simulink model "System_discrete_RST"  (R2020a)
settings: Solver=FixedStepAuto  StartTime=0.0  StopTime=30  RelTol=1e-3
values from neighbouring files (symbols this model uses):
  Te = 1e-3    (= 0.001)    [CommandeMCC.m]
undefined symbols (not defined in the file or in its folder): Amat, Bmat, ConsPolDen, ConsPolNum, RetPolDen, RetPolNum, SatPolDen, SatPolNum
libraries: simulink x1
settings Model: Creator=antoi  LastModifiedBy=antoi
settings OptimizationCC: OptimizeBlockIOStorage=off  OptimizeDataStoreBuffers=off  BusAssignmentInplaceUpdate=off
settings DebuggingCC: SFUnexpectedBacktrackingDiag=warning  SFNoUnconditionalDefaultTransitionDiag=warning
settings RTWCC: GenerateReport=on  BuildConfiguration=Debug  LaunchReport=on
settings CodeAppCC: ForceParamTrailComments=on  MATLABSourceComments=on  EnableCustomComments=on
settings GRTTargetCC: CombineSignalStateStructs=on  SupportVariableSizeSignals=on  MultiInstanceErrorCode=Warning

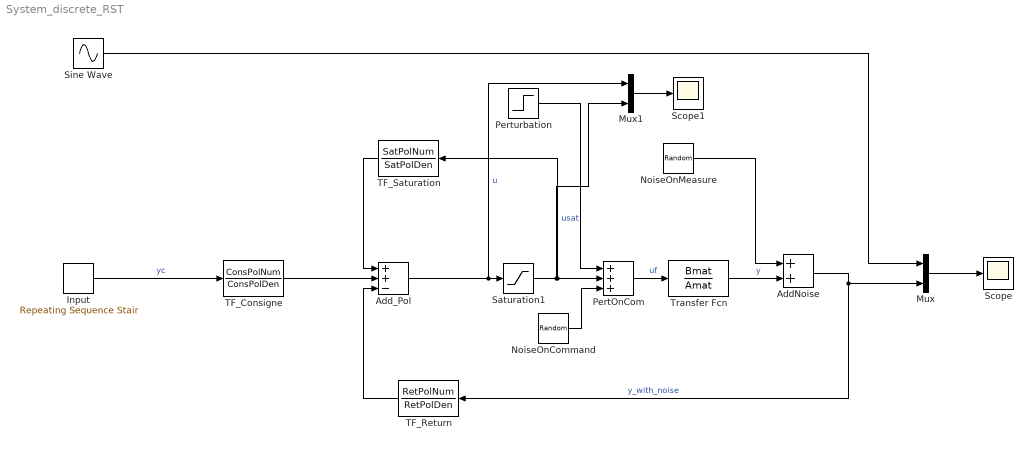
== system System_discrete_RST ==
  AddNoise : Sum
  Add_Pol : Sum  Inputs=++-
  Input : simulink/Sources/Repeating Sequence Stair  OutValues=[1 -1]'  tsamp=1  OutMin=[]  OutMax=[]  OutDataTypeStr=double  OutputDataTypeScalingMode=double  OutDataType=fixdt(0,8)  ConRadixGroup=Best Precision: Vector-wise  OutScaling=2^-12
  Mux : Mux  Inputs=2
  Mux1 : Mux  Inputs=2
  NoiseOnCommand : RandomNumber  Variance=0.01  SampleTime=0.1
  NoiseOnMeasure : RandomNumber  Variance=0.001  SampleTime=0.1
  PertOnCom : Sum  Inputs=+++
  Perturbation : Step  Time=3  After=-0.5  SampleTime=0
  Saturation1 : Saturate  UpperLimit=12  LowerLimit=-12
  Scope : Scope
  Scope1 : Scope
  Sine Wave : Sin  Frequency=6.2831853/2  Phase=pi  SampleTime=0
  TF_Consigne : DiscreteTransferFcn  Numerator=ConsPolNum  Denominator=ConsPolDen  SampleTime=Te
  TF_Return : DiscreteTransferFcn  Numerator=RetPolNum  Denominator=RetPolDen  SampleTime=Te
  TF_Saturation : DiscreteTransferFcn  Numerator=SatPolNum  Denominator=SatPolDen  SampleTime=Te
  Transfer Fcn : TransferFcn  Numerator=Bmat  Denominator=Amat
  wires:
  TF_Return/1 -> Add_Pol/3
  Add_Pol/1 -> Mux1/1, Saturation1/1  "u"
  NoiseOnMeasure/1 -> AddNoise/1
  AddNoise/1 -> TF_Return/1, Mux/2  "y_with_noise"
  Transfer Fcn/1 -> AddNoise/2  "y"
  Saturation1/1 -> Mux1/2, TF_Saturation/1, PertOnCom/2  "usat"
  Sine Wave/1 -> Mux/1
  TF_Consigne/1 -> Add_Pol/2
  PertOnCom/1 -> Transfer Fcn/1  "uf"
  Input/1 -> TF_Consigne/1  "yc"
  TF_Saturation/1 -> Add_Pol/1
  Perturbation/1 -> PertOnCom/1
  Mux/1 -> Scope/1
  NoiseOnCommand/1 -> PertOnCom/3
  Mux1/1 -> Scope1/1
